simulink model "power_aircraft_distribution"  (R2014b)
settings: Solver=ode4  StartTime=0.0  StopTime=4.5  FixedStep=Ts  RelTol=5e-3
PreLoadFcn:
  | warning off
  | Ts=10e-6;
InitFcn:
  | warning off
  | Ts=10e-6;
StopFcn:
  | warning on
undefined symbols (not defined in the file or in its folder): D1, Delta, driveGuiManager, gcbh, sigbuilder_block
libraries: powerlib x51, simulink x4, simulink_extras x4, AC6DriveInternalModels x3, powerlib_meascontrol x2, DriveInternalModels x1, sps_avr x1
(part 1 of 2)
Description:
  | Copyright 2008-2014 The MathWorks, Inc.
settings Model: FPTRunName=Active  Creator=MathWorks  LastModifiedBy=JPSOLIV
settings SolverCC: MaxOrder=2  InsertRTBMode=Auto
settings DataIOCC: LimitDataPoints=off  SignalLoggingSaveFormat=ModelDataLogs  SaveOutput=off  SaveTime=off
settings OptimizationCC: ExpressionDepthLimit=2147483647  RollThreshold=1  InitFltsAndDblsToZero=on
settings DebuggingCC: SaveWithParameterizedLinksMsg=none  UnderspecifiedInitializationDetection=Classic  MergeDetectMultiDrivingBlocksExec=none  SignalResolutionControl=TryResolveAllWithWarning  MultiTaskDSMMsg=warning  MultiTaskCondExecSysMsg=none  MultiTaskRateTransMsg=warning  FcnCallInpInsideContextMsg=UseLocalSettings  StateNameClashWarn=warning
settings HardwareCC: TargetLongLongMode=on  TargetEndianess=LittleEndian  TargetHWDeviceType=MATLAB Host  ProdEqTarget=off
settings RTWCC: IncludeERTFirstTime=on
settings GRTTargetCC: TargetFcnLib=ansi_tfl_tmw.mat  CombineOutputUpdateFcns=off  GRTInterface=on

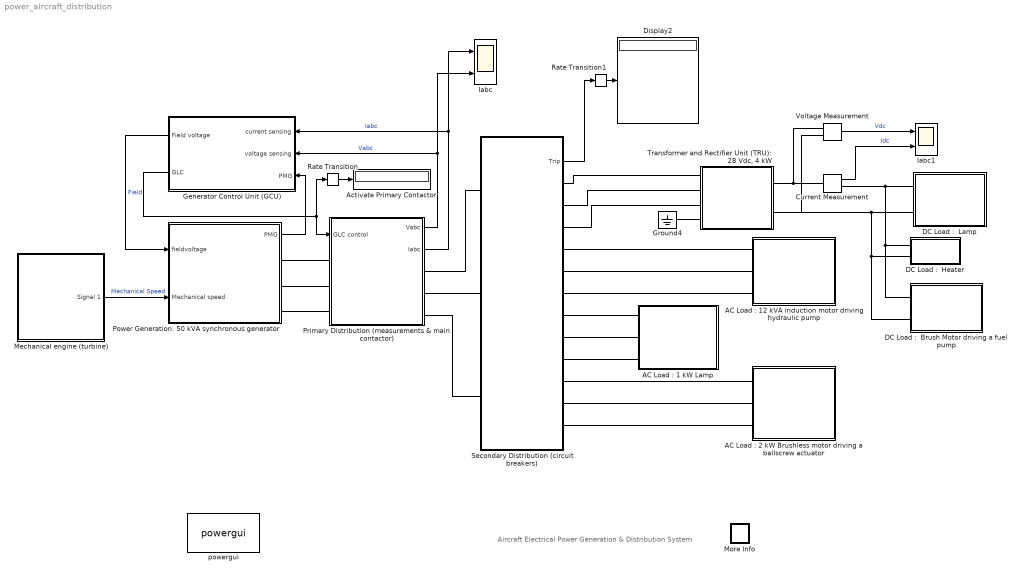
== system power_aircraft_distribution ==
  note: Aircraft Electrical Power Generation & Distribution System
  "AC Load : 1 kW Lamp" : Subsystem
      mask Display: image(imread('power_aircraft_distribution_ACLamp.jpg','jpg'))
  "AC Load : 12 kVA induction motor driving hydraulic pump" : Subsystem
      mask Display: image(imread('power_aircraft_distribution_EnginePump.jpg','jpg'))
  "AC Load : 2 kW Brushless motor driving a ballscrew actuator" : Subsystem
      mask Display: image(imread('power_aircraft_distribution_ballscrew.jpg','jpg'))
  Activate Primary Contactor : Display
      settings: SampleTime=1e-2
  Current Measurement : powerlib/Measurements/Current Measurement  PhasorSimulation=off  OutputType=Complex  PSBequivalent=0
  "DC Load :  Brush Motor driving a fuel pump" : Subsystem
      mask Display: image(imread('power_aircraft_distribution_FuelPump.jpg','jpg'))
  "DC Load :  Heater" : Subsystem
      mask Display: image(imread('power_aircraft_distribution_heater.jpg','jpg'))
  "DC Load :  Lamp" : Subsystem
      mask Display: image(imread('power_aircraft_distribution_DCLamp.jpg','jpg'))
  Display2 : Display
      settings: SampleTime=1e-2
  Generator Control Unit (GCU) : Subsystem
      mask Display: image(imread('power_aircraft_distribution_GCU.jpg','jpg'))
  Ground4 : powerlib/Elements/Ground  LConnTagsString=a
  Iabc : Scope  NumInputPorts=2
      settings: YMin=-5~-5  YMax=5~5
  Iabc1 : Scope  NumInputPorts=2
      settings: YMin=-5~-5  YMax=5~5
  Mechanical engine (turbine) : Subsystem  Tag=STV Subsys  LoadFcn=sigbuilder_block('load');  StartFcn=sigbuilder_block('start');  StopFcn=sigbuilder_block('stop');  ClipboardFcn=sigbuilder_block('clipboard');  mask(Sigbuilder block){}
      mask help: Sigbuilder GUI
      mask init:
      | if ~strcmp(get_param(bdroot(gcbh),'SimulationStatus'),'stopped') tuvar = sigbuilder_block('maskInit'); end
      settings: CopyFcn=sigbuilder_block('copy');  DeleteFcn=sigbuilder_block('delete');  ModelCloseFcn=sigbuilder_block('modelClose');  PreSaveFcn=sigbuilder_block('preSave');  PauseFcn=sigbuilder_block('pause')  ContinueFcn=sigbuilder_block('continue')  NameChangeFcn=sigbuilder_block('namechange');  OpenFcn=sigbuilder_block('open',[3 22.5 1194 819 ]);  CloseFcn=sigbuilder_block('close');
      mask Display: image(imread('power_aircraft_distribution_turbine.jpg','jpg'))
  More Info : Subsystem
      settings: OpenFcn=showdemo(bdroot(gcb))
      mask Display: disp('?')
  Power Generation: 50 kVA synchronous generator : Subsystem
      mask Display: image(imread('power_aircraft_distribution_APU_Generator.jpg','jpg'))
  Primary Distribution (measurements & main contactor) : Subsystem
  Rate Transition : RateTransition  OutPortSampleTimeOpt=Inherit  OutPortSampleTime=Ts
  Rate Transition1 : RateTransition  OutPortSampleTimeOpt=Inherit  OutPortSampleTime=Ts
  Secondary Distribution (circuit breakers) : Subsystem  mask{FuseA=25, FuseB=200, FuseC=5, FuseD=30}
      mask prompts: FuseA "Breaker  TRU (Amps RMS)"; FuseB "Breaker AC motor (Amps RMS)"; FuseC "Breaker Lamp (Amps RMS)"; FuseD "Breaker Brushless (Amps RMS)"
  "Transformer and Rectifier Unit (TRU): 28 Vdc, 4 kW" : Subsystem
      mask Display: image(imread('power_aircraft_distribution_TRU.jpg','jpg'))
  Voltage Measurement : powerlib/Measurements/Voltage Measurement  PhasorSimulation=off  OutputType=Complex  PSBequivalent=0
  powergui : powerlib/powergui  SimulationMode=Discrete  SolverType=Tustin/Backward Euler (TBE)  SampleTime=Ts  frequency=60  SPID=off  DisableSnubberDevices=off  DisableRonSwitches=off  DisableVfSwitches=off  SwTol=0  DisplayEquations=off  Interpol=off  methode=off  Ts=0  frequencyindice=0  Pbase=100e6  ErrMax=1e-4  Iterations=50  UnitsV=kV  UnitsW=MW  FunctionMessages=off  echomessages=off  HookPort=off  EnableUseOfTLC=off  x0status=blocks  RestoreLinks=no  ResistiveCurrentMeasurement=off  Frange=[0:2:500]  Ylog=off  Xlog=on  ShowGrid=off  save=off  variable=ZData  structure=0  ZoomFFT=on  StartTime=0.0  cycles=1  DisplayStyle=1  fundamental=60  FreqAxis=off  MaxFrequency=1000  frequencyindicesteady=1  RmsSteady=1  display=off
  wires:
  Power Generation: 50 kVA synchronous generator/1(PMG) -> Generator Control Unit (GCU)/3(PMG)
  Generator Control Unit (GCU)/1(Field voltage) -> Power Generation: 50 kVA synchronous generator/1(fieldvoltage)  "Field"
  Primary Distribution (measurements & main contactor)/1(Vabc) -> Generator Control Unit (GCU)/2(voltage sensing), Iabc/2  "Vabc"
  Primary Distribution (measurements & main contactor)/2(Iabc) -> Iabc/1, Generator Control Unit (GCU)/1(current sensing)  "Iabc"
  Generator Control Unit (GCU)/2(GLC) -> Primary Distribution (measurements & main contactor)/1(GLC control), Rate Transition/1
  Secondary Distribution (circuit breakers)/1(Trip) -> Rate Transition1/1
  Mechanical engine (turbine)/1(Signal 1) -> Power Generation: 50 kVA synchronous generator/2(Mechanical speed)  "Mechanical Speed"
  Current Measurement/1 -> Iabc1/2  "Idc"
  Voltage Measurement/1 -> Iabc1/1  "Vdc"
  Rate Transition/1 -> Activate Primary Contactor/1
  Rate Transition1/1 -> Display2/1
  connections:
  Power Generation: 50 kVA synchronous generator/RConn1 -- Primary Distribution (measurements & main contactor)/LConn1
  Power Generation: 50 kVA synchronous generator/RConn2 -- Primary Distribution (measurements & main contactor)/LConn2
  Power Generation: 50 kVA synchronous generator/RConn3 -- Primary Distribution (measurements & main contactor)/LConn3
  Primary Distribution (measurements & main contactor)/RConn1 -- Secondary Distribution (circuit breakers)/LConn1
  Secondary Distribution (circuit breakers)/LConn2 -- Primary Distribution (measurements & main contactor)/RConn2
  Secondary Distribution (circuit breakers)/LConn3 -- Primary Distribution (measurements & main contactor)/RConn3
  Secondary Distribution (circuit breakers)/RConn5 -- "AC Load : 12 kVA induction motor driving hydraulic pump"/LConn2
  Secondary Distribution (circuit breakers)/RConn6 -- "AC Load : 12 kVA induction motor driving hydraulic pump"/LConn3
  Secondary Distribution (circuit breakers)/RConn12 -- "AC Load : 2 kW Brushless motor driving a ballscrew actuator"/LConn3
  Secondary Distribution (circuit breakers)/RConn10 -- "AC Load : 2 kW Brushless motor driving a ballscrew actuator"/LConn1
  Secondary Distribution (circuit breakers)/RConn4 -- "AC Load : 12 kVA induction motor driving hydraulic pump"/LConn1
  Ground4/LConn1 -- "Transformer and Rectifier Unit (TRU): 28 Vdc, 4 kW"/LConn4
  Secondary Distribution (circuit breakers)/RConn11 -- "AC Load : 2 kW Brushless motor driving a ballscrew actuator"/LConn2
  "DC Load :  Lamp"/LConn1 -- "DC Load :  Heater"/LConn1 -- "DC Load :  Brush Motor driving a fuel pump"/LConn1 -- Current Measurement/RConn1
  "Transformer and Rectifier Unit (TRU): 28 Vdc, 4 kW"/RConn1 -- Current Measurement/LConn1 -- Voltage Measurement/LConn1
  "DC Load :  Heater"/LConn2 -- "DC Load :  Brush Motor driving a fuel pump"/LConn2 -- Voltage Measurement/LConn2 -- "Transformer and Rectifier Unit (TRU): 28 Vdc, 4 kW"/RConn2 -- "DC Load :  Lamp"/LConn2
  Secondary Distribution (circuit breakers)/RConn1 -- "Transformer and Rectifier Unit (TRU): 28 Vdc, 4 kW"/LConn1
  Secondary Distribution (circuit breakers)/RConn2 -- "Transformer and Rectifier Unit (TRU): 28 Vdc, 4 kW"/LConn2
  Secondary Distribution (circuit breakers)/RConn3 -- "Transformer and Rectifier Unit (TRU): 28 Vdc, 4 kW"/LConn3
  Secondary Distribution (circuit breakers)/RConn7 -- "AC Load : 1 kW Lamp"/LConn1
  Secondary Distribution (circuit breakers)/RConn8 -- "AC Load : 1 kW Lamp"/LConn2
  Secondary Distribution (circuit breakers)/RConn9 -- "AC Load : 1 kW Lamp"/LConn3

== system power_aircraft_distribution/AC Load : 1 kW Lamp ==
  note: AC Load
  Lamp 1000 Watts : powerlib/Elements/Three-Phase Series RLC Load  LConnTagsString=A|B|C  Configuration=Y (grounded)  NominalVoltage=200  NominalFrequency=400  ActivePower=1000  InductivePower=0  CapacitivePower=0  Measurements=None  LoadType=constant Z
  A : PMIOPort  Port=1  Side=Left
  B : PMIOPort  Port=2  Side=Left
  C : PMIOPort  Port=3  Side=Left
  connections:
  A/RConn1 -- Lamp 1000 Watts/LConn1
  B/RConn1 -- Lamp 1000 Watts/LConn2
  C/RConn1 -- Lamp 1000 Watts/LConn3

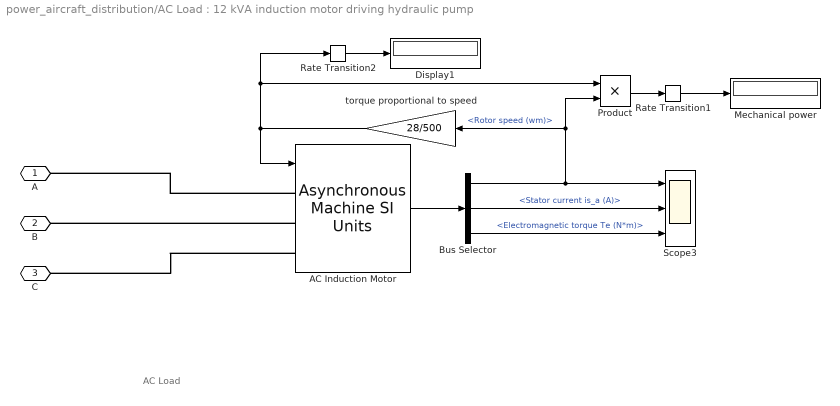
== system power_aircraft_distribution/AC Load : 12 kVA induction motor driving hydraulic pump ==
  note: AC Load
  AC Induction Motor : powerlib/Machines/Asynchronous Machine SI Units  PresetModel=No  MechanicalLoad=Torque Tm  ShowDetailedParameters=on  RotorType=Squirrel-cage  ReferenceFrame=Rotor  Units=SI  MeasurementBus=off  NominalParameters=[12e3 200 400]  Stator=[0.2761 0.002191/10]  Rotor=[0.16 0.002191/10]  Cage1=[ 0.022 0.226/377]  Cage2=[ 0.022 0.226/377]  Lm=0.07614  Mechanical=[0.01 0 8]  PolePairs=8  InitialConditions=[1,0 0,0,0 0,0,0]  SimulateSaturation=off  Saturation=[14.03593122, 27.81365428, 53.79336849, 72.68890987, 97.98006896, 148.6815601, 215.7428561, 302.9841135, 428.7778367 ; 230, 322, 414, 460, 506, 552, 598, 644, 690]  LoadFlowParameters=0  TsPowergui=0  TsBlock=-1  IterativeModel=Trapezoidal non iterative  Pmec=0
  Bus Selector : BusSelector  OutputSignals=Mechanical.Rotor speed (wm),Stator measurements.Stator current is_a (A),Mechanical.Electromagnetic torque Te (N*m)
  Display1 : Display
      settings: SampleTime=1e-2
  Mechanical power : Display
      settings: SampleTime=1e-2
  Product : Product  RndMeth=Zero
  Rate Transition1 : RateTransition  OutPortSampleTimeOpt=Inherit  OutPortSampleTime=Ts
  Rate Transition2 : RateTransition  OutPortSampleTimeOpt=Inherit  OutPortSampleTime=Ts
  Scope3 : Scope  NumInputPorts=3
  torque proportional to speed : Gain  Gain=28/500
  A : PMIOPort  Port=1  Side=Left
  B : PMIOPort  Port=2  Side=Left
  C : PMIOPort  Port=3  Side=Left
  wires:
  AC Induction Motor/1 -> Bus Selector/1
  Bus Selector/1 -> Scope3/1, torque proportional to speed/1, Product/2  "<Rotor speed (wm)>"
  torque proportional to speed/1 -> AC Induction Motor/1, Product/1, Rate Transition2/1
  Product/1 -> Rate Transition1/1
  Bus Selector/2 -> Scope3/2  "<Stator current is_a (A)>"
  Bus Selector/3 -> Scope3/3  "<Electromagnetic torque Te (N*m)>"
  Rate Transition1/1 -> Mechanical power/1
  Rate Transition2/1 -> Display1/1
  connections:
  AC Induction Motor/LConn2 -- B/RConn1
  AC Induction Motor/LConn1 -- A/RConn1
  AC Induction Motor/LConn3 -- C/RConn1

== system power_aircraft_distribution/AC Load : 2 kW Brushless motor driving a ballscrew actuator ==
  note: AC Load
  Gain : Gain  Gain=0.2
  Line inductor : powerlib/Elements/Three-Phase Series RLC Branch  LConnTagsString=A|B|C  RConnTagsString=A|B|C  BranchType=L  Resistance=[]  Inductance=1e-3  Capacitance=[]  Measurements=None
  PM Synchronous Motor Drive1 : Subsystem  LoadFcn=driveGuiManager('Load',get_param(gcb,'driveType'), gcbh);  mask(PM Synchronous Motor Drive){AverageValue=on, MechanicalLoad=Torque Tm, driveType=AC6}
      mask prompts: AverageValue "Average value model"; MechanicalLoad "Mechanical input:"; driveType "Drive type:"
      mask init:
      | block = gcbh;
      | [X1,X1m,X2,X2m,X3,X4,Y1,Y1m,Y2,Y2m,Y3,Y4,color1,color2]=spsdrivelogo;
      | Ts = drivelibInitSampleTime(block);    
      | driveGuiManager('Siminit',driveType,block);
      | SetInternalDriveModel(driveType,AverageValue,block);
      | setInternalDriveMechInput(driveType,getfullname(block));
      | power_initmask();
      settings: DeleteFcn="driveGuiManager('Delete',get_param(gcb,'driveType')  ,gcbh)"  CloseFcn="driveGuiManager('Delete',get_param(gcb,'driveType')  ,gcbh)"  ParentCloseFcn="driveGuiManager('Hide',get_param(gcb,'driveType')  ,gcbh)"
      settings: OpenFcn=|
      | if (power_openblockproxy ('secondary'))
      | driveGuiManager('Create',get_param(gcb,'driveType')  ,gcbh)
      | end;
      mask Help: helpview(psbhelp)
      mask TypeOptions MechanicalLoad: Torque Tm | Speed w
      mask TypeOptions driveType: AC6
      mask Display:
      | patch([X1 X1m],[Y1 Y1m],color1);
      | patch(X3,Y3,color2);
      | plot([X1 X1m X2 X2m X3 X4],[Y1 Y1m Y2 Y2m Y3 Y4]);
      | text(0.5,0.3,'AC6','HorizontalAlignment','center')
  Scope : Scope  NumInputPorts=4
  Speed : powerlib_meascontrol/Pulse & Signal Generators/Stair Generator  t=[0 1.4 1.9 2.4 3]  e=[0 500 0 -500 0]  Ts=Ts
  demux : Subsystem
  A : PMIOPort  Port=1  Side=Left
  B : PMIOPort  Port=2  Side=Left
  C : PMIOPort  Port=3  Side=Left
  wires:
  Speed/1 -> PM Synchronous Motor Drive1/1(SP)
  Gain/1 -> PM Synchronous Motor Drive1/2(Tm)
  demux/1(i_a) -> Scope/1  "Stator current"
  demux/2(speed) -> Scope/2  "Rotor speed"
  demux/3(Tem) -> Scope/3  "Electromagnetic Torque"
  demux/4(v_dc) -> Scope/4  "DC bus voltage"
  PM Synchronous Motor Drive1/4(Wm) -> Gain/1
  PM Synchronous Motor Drive1/1(Motor) -> demux/1(motor)
  PM Synchronous Motor Drive1/2(Conv.) -> demux/2(Conv.)
  PM Synchronous Motor Drive1/3(Ctrl) -> demux/3(Ctrl)
  connections:
  Line inductor/RConn3 -- PM Synchronous Motor Drive1/LConn3
  Line inductor/RConn2 -- PM Synchronous Motor Drive1/LConn2
  Line inductor/RConn1 -- PM Synchronous Motor Drive1/LConn1
  Line inductor/LConn3 -- C/RConn1
  Line inductor/LConn2 -- B/RConn1
  Line inductor/LConn1 -- A/RConn1

== system power_aircraft_distribution/DC Load :  Brush Motor driving a fuel pump ==
  note: DC Load
  Bus Selector : BusSelector  OutputSignals=Speed wm (rad/s),Armature current ia (A),Electrical torque Te (n m)
  DC Machine : powerlib/Machines/DC Machine  PresetModel=No  MechanicalLoad=Torque TL  FieldType=Wound  ShowDetailedParameters=on  MeasurementBus=off  RLa=[ .35 0.0001]  RLf="[ 240  12]"  Laf=1  MachineConstant=Torque constant (N.m/A)  Ke=1.8  Kt=1.8  J=0.0005  Bm=0  Tf=0  w0=0  Ifinit=0  TsPowergui=0  TsBlock=-1
  Gain : Gain  Gain=1.5/200
  Scope3 : Scope  NumInputPorts=3
  + : PMIOPort  Port=1  Side=Left
  - : PMIOPort  Port=2  Side=Left
  wires:
  Gain/1 -> DC Machine/1
  DC Machine/1 -> Bus Selector/1
  Bus Selector/1 -> Scope3/1, Gain/1  "<Speed wm (rad/s)>"
  Bus Selector/2 -> Scope3/2  "<Armature current ia (A)>"
  Bus Selector/3 -> Scope3/3  "<Electrical torque Te (n m)>"
  connections:
  -/RConn1 -- DC Machine/RConn1 -- DC Machine/RConn2
  +/RConn1 -- DC Machine/LConn1 -- DC Machine/LConn2

== system power_aircraft_distribution/DC Load :  Heater ==
  note: DC Load
  Series RLC Branch3 : powerlib/Elements/Series RLC Branch  LConnTagsString=__new0  RConnTagsString=__new0  BranchType=R  Resistance=1  Inductance=[]  SetiL0=off  InitialCurrent=0  Capacitance=[]  Setx0=off  InitialVoltage=0  Measurements=Branch voltage and current
  + : PMIOPort  Port=1  Side=Left
  - : PMIOPort  Port=2  Side=Left
  connections:
  -/RConn1 -- Series RLC Branch3/RConn1
  +/RConn1 -- Series RLC Branch3/LConn1

== system power_aircraft_distribution/DC Load :  Lamp ==
  note: DC Load
  Series RLC Branch3 : powerlib/Elements/Series RLC Branch  LConnTagsString=__new0  RConnTagsString=__new0  BranchType=R  Resistance=1  Inductance=[]  SetiL0=off  InitialCurrent=0  Capacitance=[]  Setx0=off  InitialVoltage=0  Measurements=Branch voltage and current
  + : PMIOPort  Port=1  Side=Left
  - : PMIOPort  Port=2  Side=Left
  connections:
  +/RConn1 -- Series RLC Branch3/LConn1
  -/RConn1 -- Series RLC Branch3/RConn1

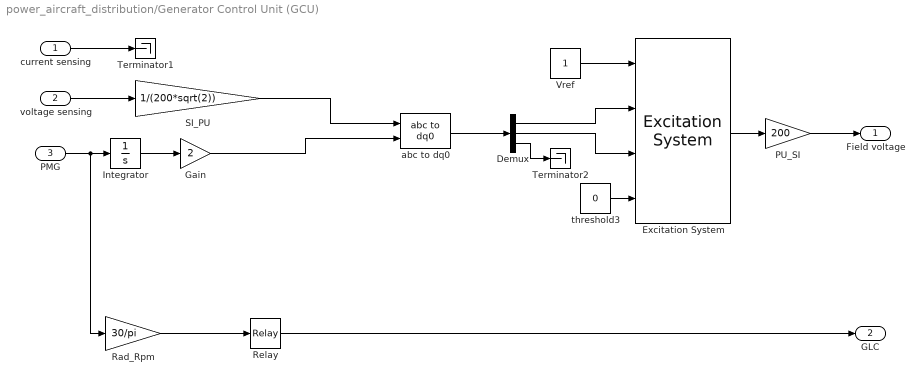
== system power_aircraft_distribution/Generator Control Unit (GCU) ==
  current sensing : Inport
  voltage sensing : Inport  Port=2
  PMG : Inport  Port=3
  Demux : Demux  Outputs=3
  Excitation System : sps_avr/Excitation System  tr=20e-3  reg=[ 300, 0.001 ]  exc=[ 1, 0 ]  tgr=[ 0, 0 ]  damp=[ 0.001, 0.1 ]  sat=[ 0, 0 ]  lim=[ -2, 2, 0 ]  v0=[1 0]
  Gain : Gain  Gain=2
  Integrator : Integrator
  PU_SI : Gain  Gain=200
  Rad_Rpm : Gain  Gain=30/pi
  Relay : Relay  OnSwitchValue=9000  OffSwitchValue=8900
  SI_PU : Gain  Gain=1/(200*sqrt(2))
  Terminator1 : Terminator
  Terminator2 : Terminator
  Vref : Constant
  abc to dq0 : powerlib_meascontrol/Transformations/abc to dq0  Alignment=90 degrees behind phase A axis
  threshold3 : Constant  Value=0
  Field voltage : Outport
  GLC : Outport  Port=2
  wires:
  Relay/1 -> GLC/1
  Demux/3 -> Terminator2/1
  current sensing/1 -> Terminator1/1
  threshold3/1 -> Excitation System/4
  Vref/1 -> Excitation System/1
  Rad_Rpm/1 -> Relay/1
  PU_SI/1 -> Field voltage/1
  Excitation System/1 -> PU_SI/1
  SI_PU/1 -> abc to dq0/1
  Demux/2 -> Excitation System/3
  Demux/1 -> Excitation System/2
  abc to dq0/1 -> Demux/1
  Integrator/1 -> Gain/1
  voltage sensing/1 -> SI_PU/1
  PMG/1 -> Rad_Rpm/1, Integrator/1
  Gain/1 -> abc to dq0/2

== system power_aircraft_distribution/Mechanical engine (turbine) ==
  Demux : Demux  Tag=STV Demux  Outputs=1
  FromWs : FromWorkspace  Tag=STV FromWs  VariableName=tuvar  SampleTime=0
      SigBuilderData=|
      | common.afterFinalStr = 'Extrapolate'
      | common.sampleTime = 0
      | dataSet.timeRange = [0 10]
      | dataSet.name = 'Group 1'
      | sbobj.Groups.Name = 'Group 1'
      | sbobj.Groups.Signals.Name = 'Signal 1'
      | sbobj.Groups.Signals.XData = [0 0.4 0.5 1 2 3 4.5 6 6 10]
      | sbobj.Groups.Signals.YData = [0 12000 12000 12000 12000 10000 18000 1 0 0]
  Signal 1 : Outport  Tag=STV Outport
  wires:
  FromWs/1 -> Demux/1
  Demux/1 -> Signal 1/1

== system power_aircraft_distribution/More Info ==

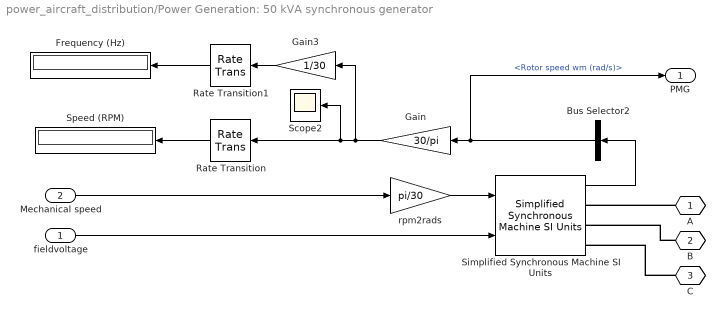
== system power_aircraft_distribution/Power Generation: 50 kVA synchronous generator ==
  fieldvoltage : Inport
  Mechanical speed : Inport  Port=2
  Bus Selector2 : BusSelector  OutputSignals=Rotor speed wm (rad/s)
  Frequency (Hz) : Display
      settings: SampleTime=1e-2
  Gain : Gain  Gain=30/pi
  Gain3 : Gain  Gain=1/30
  Rate Transition : RateTransition  OutPortSampleTimeOpt=Inherit  OutPortSampleTime=Ts
  Rate Transition1 : RateTransition  OutPortSampleTimeOpt=Inherit  OutPortSampleTime=Ts
  Scope2 : Scope
  Simplified Synchronous Machine SI Units : powerlib/Machines/Simplified Synchronous Machine SI Units  ConnectionType=3-wire Y  MechanicalLoad=Speed w  MeasurementBus=off  NominalParameters=[50e3 200 400]  Mechanical=[0.02 0 2]  InternalRL="[0.0204  0.08104e-3]"  InitialConditions=[-99,0 0,0,0 0,0,0]  Units=1  LoadFlowParameters=[1,0,0,0,0]  TsPowergui=0  TsBlock=Ts  BusType=PV  Pref=0  Qref=0  Qmin=-inf  Qmax=+inf  PLF=0  QLF=0
  Speed (RPM) : Display
      settings: SampleTime=1e-2
  rpm2rads : Gain  Gain=pi/30
  A : PMIOPort  Tag=PMCPort  Port=1  Side=Right
  B : PMIOPort  Tag=PMCPort  Port=2  Side=Right
  C : PMIOPort  Tag=PMCPort  Port=3  Side=Right
  PMG : Outport
  wires:
  Simplified Synchronous Machine SI Units/1 -> Bus Selector2/1
  fieldvoltage/1 -> Simplified Synchronous Machine SI Units/2
  Bus Selector2/1 -> Gain/1, PMG/1  "<Rotor speed wm (rad/s)>"
  Gain/1 -> Gain3/1, Scope2/1, Rate Transition/1
  Gain3/1 -> Rate Transition1/1
  Mechanical speed/1 -> rpm2rads/1
  rpm2rads/1 -> Simplified Synchronous Machine SI Units/1
  Rate Transition/1 -> Speed (RPM)/1
  Rate Transition1/1 -> Frequency (Hz)/1
  connections:
  A/RConn1 -- Simplified Synchronous Machine SI Units/RConn1
  B/RConn1 -- Simplified Synchronous Machine SI Units/RConn2
  C/RConn1 -- Simplified Synchronous Machine SI Units/RConn3

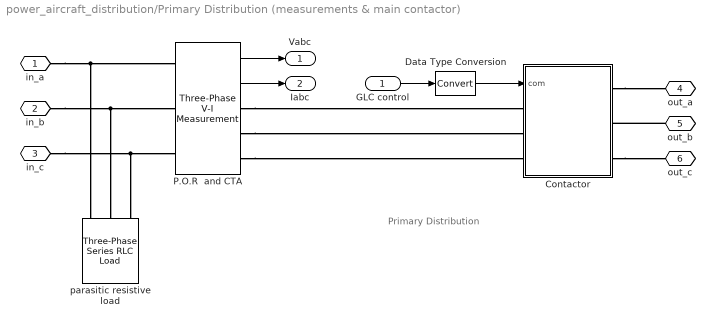
== system power_aircraft_distribution/Primary Distribution (measurements & main contactor) ==
  note: Primary Distribution
  GLC control : Inport
  Contactor : Subsystem
  Data Type Conversion : DataTypeConversion
  P.O.R  and CTA : powerlib/Measurements/Three-Phase V-I Measurement  VoltageMeasurement=phase-to-phase  SetLabelV=off  LabelV=Vabc  Vpu=off  VpuLL=off  CurrentMeasurement=yes  SetLabelI=off  LabelI=Iabc  Ipu=off  Pbase=100e6  Vbase=500e3  OutputType=Complex  PhasorSimulation=off  PSBequivalent=0
  parasitic resistive load : powerlib/Elements/Three-Phase Series RLC Load  LConnTagsString=A|B|C  Configuration=Y (grounded)  NominalVoltage=200  NominalFrequency=400  ActivePower=5000  InductivePower=0  CapacitivePower=0  Measurements=None  LoadType=constant Z
  in_a : PMIOPort  Port=1  Side=Left
  in_b : PMIOPort  Port=2  Side=Left
  in_c : PMIOPort  Port=3  Side=Left
  out_a : PMIOPort  Port=4  Side=Right
  out_b : PMIOPort  Port=5  Side=Right
  out_c : PMIOPort  Port=6  Side=Right
  Vabc : Outport
  Iabc : Outport  Port=2
  wires:
  GLC control/1 -> Data Type Conversion/1
  P.O.R  and CTA/1 -> Vabc/1
  P.O.R  and CTA/2 -> Iabc/1
  Data Type Conversion/1 -> Contactor/1(com)
  connections:
  in_a/RConn1 -- P.O.R  and CTA/LConn1 -- parasitic resistive load/LConn1
  in_b/RConn1 -- P.O.R  and CTA/LConn2 -- parasitic resistive load/LConn2
  in_c/RConn1 -- P.O.R  and CTA/LConn3 -- parasitic resistive load/LConn3
  P.O.R  and CTA/RConn1 -- Contactor/LConn1
  P.O.R  and CTA/RConn2 -- Contactor/LConn2
  P.O.R  and CTA/RConn3 -- Contactor/LConn3
  Contactor/RConn1 -- out_a/RConn1
  out_b/RConn1 -- Contactor/RConn2
  Contactor/RConn3 -- out_c/RConn1

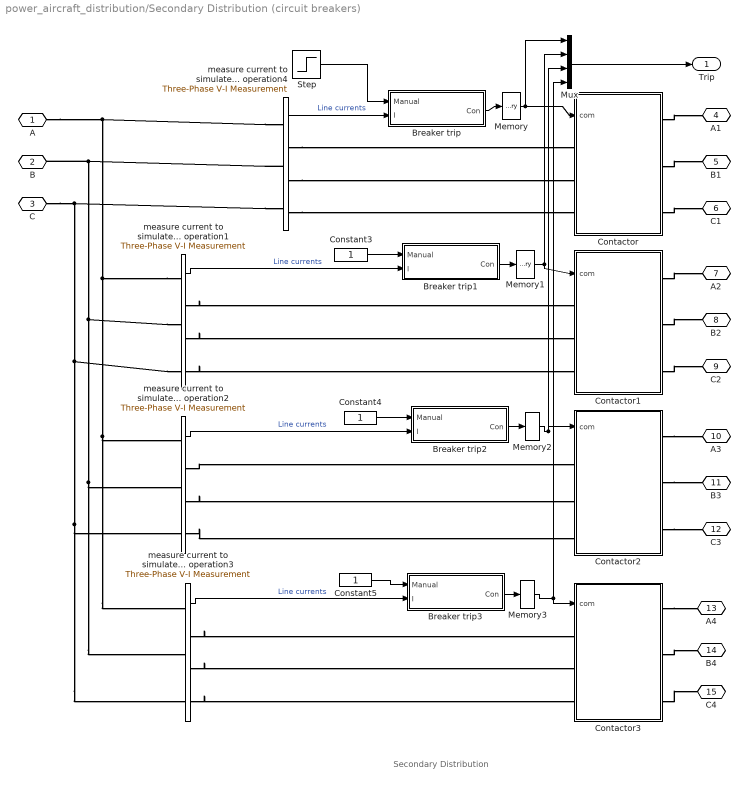
== system power_aircraft_distribution/Secondary Distribution (circuit breakers) ==
  note: Secondary Distribution
  Breaker trip : Subsystem
  Breaker trip1 : Subsystem
  Breaker trip2 : Subsystem
  Breaker trip3 : Subsystem
  Constant3 : Constant  OutDataTypeStr=boolean
  Constant4 : Constant  OutDataTypeStr=boolean
  Constant5 : Constant  OutDataTypeStr=boolean
  Contactor : Subsystem
  Contactor1 : Subsystem
  Contactor2 : Subsystem
  Contactor3 : Subsystem
  Memory{,1..3} (4 alike) : Memory
  Mux : Mux
  Step : Step  Time=3.5  Before=1  After=0  SampleTime=0
  measure current to simulate fuse operation{1..4} (4 alike) : powerlib/Measurements/Three-Phase V-I Measurement  VoltageMeasurement=no  SetLabelV=off  LabelV=Vabc  Vpu=off  VpuLL=off  CurrentMeasurement=yes  SetLabelI=off  LabelI=Iabc  Ipu=off  Pbase=100e6  Vbase=500e3  OutputType=Complex  PhasorSimulation=off  PSBequivalent=0
  A : PMIOPort  Port=1  Side=Left
  B : PMIOPort  Port=2  Side=Left
  C : PMIOPort  Port=3  Side=Left
  A1 : PMIOPort  Port=4  Side=Right
  B1 : PMIOPort  Port=5  Side=Right
  C1 : PMIOPort  Port=6  Side=Right
  A2 : PMIOPort  Port=7  Side=Right
  B2 : PMIOPort  Port=8  Side=Right
  C2 : PMIOPort  Port=9  Side=Right
  A3 : PMIOPort  Port=10  Side=Right
  B3 : PMIOPort  Port=11  Side=Right
  C3 : PMIOPort  Port=12  Side=Right
  A4 : PMIOPort  Port=13  Side=Right
  B4 : PMIOPort  Port=14  Side=Right
  C4 : PMIOPort  Port=15  Side=Right
  Trip : Outport
  wires:
  Constant3/1 -> Breaker trip1/1(Manual)
  Step/1 -> Breaker trip/1(Manual)
  Memory3/1 -> Contactor3/1(com), Mux/4
  Memory2/1 -> Contactor2/1(com), Mux/3
  Breaker trip1/1(Con) -> Memory1/1
  Memory/1 -> Contactor/1(com), Mux/1
  Memory1/1 -> Contactor1/1(com), Mux/2
  Mux/1 -> Trip/1
  Breaker trip2/1(Con) -> Memory2/1
  Breaker trip3/1(Con) -> Memory3/1
  Constant4/1 -> Breaker trip2/1(Manual)
  Constant5/1 -> Breaker trip3/1(Manual)
  measure current to simulate fuse operation3/1 -> Breaker trip3/2(I)  "Line currents"
  measure current to simulate fuse operation2/1 -> Breaker trip2/2(I)  "Line currents"
  measure current to simulate fuse operation1/1 -> Breaker trip1/2(I)  "Line currents"
  Breaker trip/1(Con) -> Memory/1
  measure current to simulate fuse operation4/1 -> Breaker trip/2(I)  "Line currents"
  connections:
  measure current to simulate fuse operation3/RConn3 -- Contactor3/LConn3
  measure current to simulate fuse operation3/RConn2 -- Contactor3/LConn2
  measure current to simulate fuse operation3/RConn1 -- Contactor3/LConn1
  Contactor3/RConn3 -- C4/RConn1
  Contactor3/RConn2 -- B4/RConn1
  Contactor3/RConn1 -- A4/RConn1
  measure current to simulate fuse operation2/RConn3 -- Contactor2/LConn3
  measure current to simulate fuse operation2/RConn2 -- Contactor2/LConn2
  measure current to simulate fuse operation2/RConn1 -- Contactor2/LConn1
  Contactor2/RConn3 -- C3/RConn1
  Contactor2/RConn2 -- B3/RConn1
  Contactor2/RConn1 -- A3/RConn1
  measure current to simulate fuse operation1/RConn3 -- Contactor1/LConn3
  measure current to simulate fuse operation1/RConn2 -- Contactor1/LConn2
  measure current to simulate fuse operation1/RConn1 -- Contactor1/LConn1
  Contactor1/RConn3 -- C2/RConn1
  Contactor1/RConn2 -- B2/RConn1
  Contactor1/RConn1 -- A2/RConn1
  measure current to simulate fuse operation4/RConn3 -- Contactor/LConn3
  measure current to simulate fuse operation4/RConn2 -- Contactor/LConn2
  measure current to simulate fuse operation4/RConn1 -- Contactor/LConn1
  Contactor/RConn3 -- C1/RConn1
  Contactor/RConn2 -- B1/RConn1
  Contactor/RConn1 -- A1/RConn1
  measure current to simulate fuse operation1/LConn3 -- measure current to simulate fuse operation4/LConn3 -- C/RConn1 -- measure current to simulate fuse operation2/LConn3 -- measure current to simulate fuse operation3/LConn3
  measure current to simulate fuse operation1/LConn2 -- measure current to simulate fuse operation2/LConn2 -- measure current to simulate fuse operation3/LConn2 -- B/RConn1 -- measure current to simulate fuse operation4/LConn2
  measure current to simulate fuse operation1/LConn1 -- measure current to simulate fuse operation2/LConn1 -- measure current to simulate fuse operation3/LConn1 -- measure current to simulate fuse operation4/LConn1 -- A/RConn1

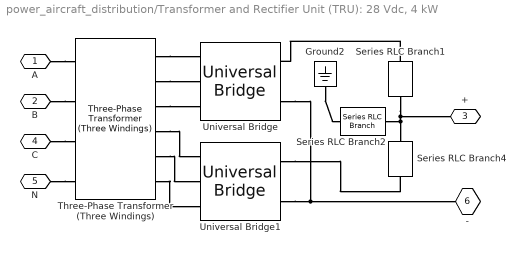
== system power_aircraft_distribution/Transformer and Rectifier Unit (TRU): 28 Vdc, 4 kW ==
  Ground2 : powerlib/Elements/Ground  LConnTagsString=a
  Series RLC Branch1 : powerlib/Elements/Series RLC Branch  LConnTagsString=__new0  RConnTagsString=__new0  BranchType=L  Resistance=[]  Inductance=2e-3  SetiL0=on  InitialCurrent=0  Capacitance=[]  Setx0=off  InitialVoltage=0  Measurements=Branch voltage and current
  Series RLC Branch2 : powerlib/Elements/Series RLC Branch  LConnTagsString=__new0  RConnTagsString=__new0  BranchType=C  Resistance=[]  Inductance=[]  SetiL0=off  InitialCurrent=0  Capacitance=1e-6  Setx0=off  InitialVoltage=0  Measurements=None
  Series RLC Branch4 : powerlib/Elements/Series RLC Branch  LConnTagsString=__new0  RConnTagsString=__new0  BranchType=L  Resistance=[]  Inductance=2e-3  SetiL0=off  InitialCurrent=0  Capacitance=[]  Setx0=off  InitialVoltage=0  Measurements=Branch voltage and current
  Three-Phase Transformer (Three Windings) : powerlib/Elements/Three-Phase Transformer (Three Windings)  Winding1Connection=Yn  UNITS=pu  NominalPower=[ 4200 , 600 ]  Winding1=[ 200 , 0.0002 , 0 ]  Winding2Connection=Delta (D1)  Winding2=[ 22 , 0.0002 , 0 ]  Winding3Connection=Delta (D1)  Winding3=[ 22 , 0.0002 , 0]  SetSaturation=off  Rm=500  Lm=500*10  Saturation=[ 0,0 ; 0.0024,1.2 ; 1.0,1.52 ]  Hysteresis=off  DataFile='hysteresis'  SetInitialFlux=off  InitialFluxes=[0.8 -0.8 0.7]  Measurements=None  MoreParameters=off  BreakLoop=off  DataType=off  TransfoNumber=0
  Universal Bridge : powerlib/Power Electronics/Universal Bridge  Arms=3  SnubberResistance=1e3  SnubberCapacitance=1e-6  Device=Diodes  Ron=1e-3  Lon=0  ForwardVoltages="[  0  0  ]"  ForwardVoltage=0.8  GTOparameters=[ 10e-6 , 20e-6 ]  IGBTparameters=[ 1e-6 , 2e-6 ]  Measurements=None  Measurements_2=None  converterType=Rectifier
  Universal Bridge1 : powerlib/Power Electronics/Universal Bridge  Arms=3  SnubberResistance=1e3  SnubberCapacitance=1e-6  Device=Diodes  Ron=1e-3  Lon=0  ForwardVoltages="[  0  0  ]"  ForwardVoltage=0.8  GTOparameters=[ 10e-6 , 20e-6 ]  IGBTparameters=[ 1e-6 , 2e-6 ]  Measurements=None  Measurements_2=None  converterType=Rectifier
  A : PMIOPort  Port=1  Side=Left
  B : PMIOPort  Port=2  Side=Left
  + : PMIOPort  Port=3  Side=Right
  C : PMIOPort  Port=4  Side=Left
  N : PMIOPort  Port=5  Side=Left
  - : PMIOPort  Port=6  Side=Right
  connections:
  Ground2/LConn1 -- Series RLC Branch2/RConn1
  Universal Bridge/RConn2 -- Universal Bridge1/RConn2 -- -/RConn1
  Three-Phase Transformer (Three Windings)/RConn1 -- Universal Bridge/LConn1
  Three-Phase Transformer (Three Windings)/RConn2 -- Universal Bridge/LConn2
  Three-Phase Transformer (Three Windings)/RConn3 -- Universal Bridge/LConn3
  A/RConn1 -- Three-Phase Transformer (Three Windings)/LConn1
  B/RConn1 -- Three-Phase Transformer (Three Windings)/LConn2
  C/RConn1 -- Three-Phase Transformer (Three Windings)/LConn3
  N/RConn1 -- Three-Phase Transformer (Three Windings)/LConn4
  Series RLC Branch1/LConn1 -- Universal Bridge/RConn1
  Series RLC Branch2/LConn1 -- Series RLC Branch1/RConn1 -- +/RConn1 -- Series RLC Branch4/LConn1
  Three-Phase Transformer (Three Windings)/RConn4 -- Universal Bridge1/LConn1
  Three-Phase Transformer (Three Windings)/RConn5 -- Universal Bridge1/LConn2
  Three-Phase Transformer (Three Windings)/RConn6 -- Universal Bridge1/LConn3
  Universal Bridge1/RConn1 -- Series RLC Branch4/RConn1

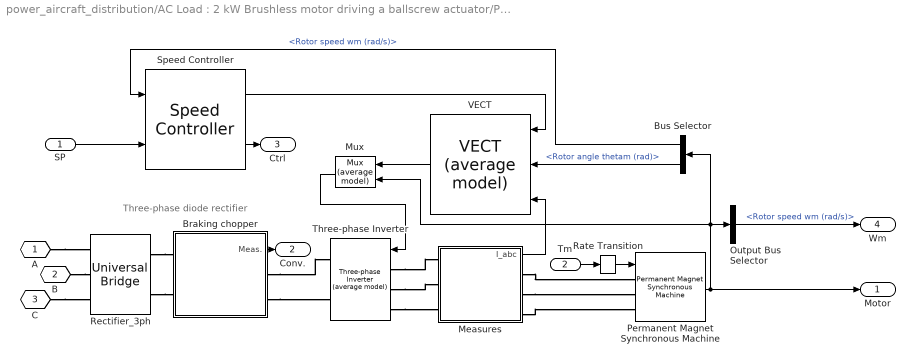
== system power_aircraft_distribution/AC Load : 2 kW Brushless motor driving a ballscrew actuator/PM Synchronous Motor Drive1 ==
  note: Three-phase
      | diode rectifier
  SP : Inport
  Tm : Inport  Port=2
  Braking chopper : Subsystem  StartFcn=|  mask(Braking chopper){chopa=290, chopd=280, freq_chop=4000, cap_bus=2000e-6, br=8}
      | chopa=str2num(get_param(gcb,'chopa'));                                                               
      | chopd=str2num(get_param(gcb,'chopd'));                                                               
      | if (chopa < chopd)                                                                                   
      |     error('Activation voltage must be greater than or equal to shutdown voltage in Braking chopper');
      | end
      mask prompts: chopa "Chopper activation voltage (V)"; chopd "Chopper shutdown voltage (V)"; freq_chop "Braking chopper frequency (Hz)"; cap_bus "DC bus capacitance (F)"; br "Braking resistance (ohms)"
      mask help: This block implement a DC link between the rectifier and the inverter. It also contains a DC bus integrated braking chopper. The braking resistor must be set properly to avoid oscillation.
      mask init:
      | if chopa < chopd;
      |     chopa = chopd;
      | end
      | [X1,X1m,X2,X2m,X3,X4,Y1,Y1m,Y2,Y2m,Y3,Y4,color1,color2]=spsdrivelogo;
      mask Display:
      | patch([X1 X1m],[Y1 Y1m],color1);
      | patch(X3,Y3,color2);
      | plot([X1 X1m X2 X2m X3 X4],[Y1 Y1m Y2 Y2m Y3 Y4]);
  Bus Selector : BusSelector  OutputSignals=Rotor speed wm (rad/s),Rotor angle thetam (rad)
  Measures : Subsystem
  Mux : AC6DriveInternalModels/Mux (average model)
  Output Bus Selector : BusSelector  OutputSignals=Rotor speed wm (rad/s)
  Permanent Magnet Synchronous Machine : powerlib/Machines/Permanent Magnet Synchronous Machine  NbPhases=3  FluxDistribution=Sinusoidal  RotorType=Round  MechanicalLoad=Torque Tm  PresetModel=No  ShowDetailedParameters=on  MeasurementBus=off  Resistance=0.2  Inductance=0  dqInductances=[8.5e-3,8.5e-3]  La=0.000835  MachineConstant=Flux linkage established by magnets (V.s)  Flux=0.175  VoltageCst=126.966  TorqueCst=1.05  Flat=0  Mechanical=[0.089,0.005,4]  PolePairs=4  InitialConditions=[0,0,0,0]  InitialConditions5ph=[0 0 0 0 0 0]  TsPowergui=0  TsBlock=-1  RefAngle=90 degrees behind phase A axis (modified Park)
      settings: AttributesFormatString=\n
  Rate Transition : RateTransition  OutPortSampleTime=Ts
  Rectifier_3ph : powerlib/Power Electronics/Universal Bridge  Arms=3  SnubberResistance=10e3  SnubberCapacitance=20e-9  Device=Diodes  Ron=1e-3  Lon=0  ForwardVoltages="[  0,  0  ]"  ForwardVoltage=1.3  GTOparameters=[ 10e-6, 20e-6 ]  IGBTparameters=[ 1e-6 , 2e-6 ]  Measurements=All voltages and currents  Measurements_2=None  converterType=Rectifier
  Speed Controller : DriveInternalModels/AC drives/Speed Controller AC67/Speed Controller  SwK=Speed regulation  ramp=[-1000,1000]  kp=5  ki=100  fc=100  ctrl_sat=[-50,50]  Tsc=150e-6
  Three-phase Inverter : AC6DriveInternalModels/Three-phase Inverter (average model)  Arms=3  SnubberResistance=5000  SnubberCapacitance=inf  Device=IGBT / Diodes  Ron=1e-3  Lon=0  ForwardVoltages=[0.8,0.8]  ForwardVoltage=0  GTOparameters=[0,0]  IGBTparameters=[1e-6,2e-6]  Measurements=All voltages and currents  converterType=Inverter  SourceFrequency=60  dqInductances=[8.5e-3,8.5e-3]  Flux=0.175  Resistance=0.2  p=4
  VECT : AC6DriveInternalModels/VECT (average model)  nb_p=4  lambda=0.175  freq_max=20e3  Ts_vect=50e-6  h=0.1
  A : PMIOPort  Port=1  Side=Left
  B : PMIOPort  Port=2  Side=Left
  C : PMIOPort  Tag=PMCPort  Port=3  Side=Left
  Motor : Outport
  Conv. : Outport  Port=2
  Ctrl : Outport  Port=3
  Wm : Outport  Port=4
  wires:
  Bus Selector/2 -> VECT/2  "<Rotor angle thetam (rad)>"
  Bus Selector/1 -> Speed Controller/1  "<Rotor speed wm (rad/s)>"
  Mux/1 -> Three-phase Inverter/1
  VECT/1 -> Mux/1
  Speed Controller/2 -> Ctrl/1
  Tm/1 -> Rate Transition/1
  Speed Controller/1 -> VECT/1
  Measures/1(I_abc) -> VECT/3
  Permanent Magnet Synchronous Machine/1 -> Output Bus Selector/1, Bus Selector/1, Mux/2, Motor/1
  SP/1 -> Speed Controller/2
  Braking chopper/1(Meas.) -> Conv./1
  Output Bus Selector/1 -> Wm/1  "<Rotor speed wm (rad/s)>"
  Rate Transition/1 -> Permanent Magnet Synchronous Machine/1
  connections:
  Three-phase Inverter/LConn3 -- Measures/LConn3
  Three-phase Inverter/LConn2 -- Measures/LConn2
  Three-phase Inverter/LConn1 -- Measures/LConn1
  C/RConn1 -- Rectifier_3ph/LConn3
  B/RConn1 -- Rectifier_3ph/LConn2
  Measures/RConn3 -- Permanent Magnet Synchronous Machine/LConn3
  Measures/RConn2 -- Permanent Magnet Synchronous Machine/LConn2
  Measures/RConn1 -- Permanent Magnet Synchronous Machine/LConn1
  Braking chopper/RConn2 -- Three-phase Inverter/RConn2
  A/RConn1 -- Rectifier_3ph/LConn1
  Rectifier_3ph/RConn1 -- Braking chopper/LConn1
  Rectifier_3ph/RConn2 -- Braking chopper/LConn2
  Braking chopper/RConn1 -- Three-phase Inverter/RConn1

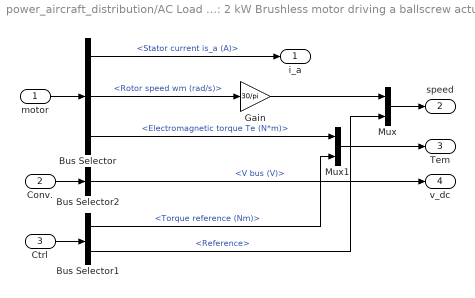
== system power_aircraft_distribution/AC Load : 2 kW Brushless motor driving a ballscrew actuator/demux ==
  motor : Inport
  Conv. : Inport  Port=2
  Ctrl : Inport  Port=3
  Bus Selector : BusSelector  OutputSignals=Stator current is_a (A),Rotor speed wm (rad/s),Electromagnetic torque Te (N*m)
  Bus Selector1 : BusSelector  OutputSignals=Torque reference (Nm),Reference
  Bus Selector2 : BusSelector  OutputSignals=V bus (V)
  Gain : Gain  Gain=30/pi  SaturateOnIntegerOverflow=on  OutDataTypeStr=Inherit: Same as input  ParamDataTypeStr=Inherit: Same as input
  Mux : Mux  Inputs=2
  Mux1 : Mux  Inputs=2
  i_a : Outport
  speed : Outport  Port=2
  Tem : Outport  Port=3
  v_dc : Outport  Port=4
  wires:
  Bus Selector/2 -> Gain/1  "<Rotor speed wm (rad/s)>"
  Bus Selector2/1 -> v_dc/1  "<V bus (V)>"
  Conv./1 -> Bus Selector2/1
  Ctrl/1 -> Bus Selector1/1
  Bus Selector1/1 -> Mux1/2  "<Torque reference (Nm)>"
  Bus Selector1/2 -> Mux/2  "<Reference>"
  Gain/1 -> Mux/1
  Bus Selector/1 -> i_a/1  "<Stator current is_a (A)>"
  Bus Selector/3 -> Mux1/1  "<Electromagnetic torque Te (N*m)>"
  Mux1/1 -> Tem/1
  Mux/1 -> speed/1
  motor/1 -> Bus Selector/1

== system power_aircraft_distribution/Primary Distribution (measurements & main contactor)/Contactor ==
  com : Inport
  Ideal Switch : powerlib/Power Electronics/Ideal Switch  Ron=0.001  Lon=0  IC=0  Rs=1e3  Cs=inf  Measurements=off
  Ideal Switch1 : powerlib/Power Electronics/Ideal Switch  Ron=0.001  Lon=0  IC=0  Rs=1e3  Cs=inf  Measurements=off
  Ideal Switch2 : powerlib/Power Electronics/Ideal Switch  Ron=0.001  Lon=0  IC=0  Rs=1e3  Cs=inf  Measurements=off
  A : PMIOPort  Port=1  Side=Left
  a : PMIOPort  Port=2  Side=Right
  B : PMIOPort  Port=3  Side=Left
  b : PMIOPort  Port=4  Side=Right
  C : PMIOPort  Port=5  Side=Left
  c : PMIOPort  Port=6  Side=Right
  wires:
  com/1 -> Ideal Switch1/1, Ideal Switch2/1, Ideal Switch/1
  connections:
  c/RConn1 -- Ideal Switch2/RConn1
  C/RConn1 -- Ideal Switch2/LConn1
  b/RConn1 -- Ideal Switch1/RConn1
  B/RConn1 -- Ideal Switch1/LConn1
  a/RConn1 -- Ideal Switch/RConn1
  A/RConn1 -- Ideal Switch/LConn1

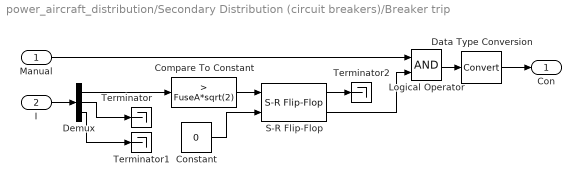
== system power_aircraft_distribution/Secondary Distribution (circuit breakers)/Breaker trip ==
  Manual : Inport
  I : Inport  Port=2
  Compare To Constant : simulink/Logic and Bit Operations/Compare To Constant  relop=>  const=FuseA*sqrt(2)  OutDataTypeStr=boolean  ZeroCross=off
  Constant : Constant  Value=0  OutDataTypeStr=boolean
  Data Type Conversion : DataTypeConversion
  Demux : Demux  Outputs=3
  Logical Operator : Logic  AllPortsSameDT=off  OutDataTypeStr=boolean
  S-R Flip-Flop : simulink_extras/Flip Flops/S-R Flip-Flop  initial_condition=0
  Terminator : Terminator
  Terminator1 : Terminator
  Terminator2 : Terminator
  Con : Outport
  wires:
  S-R Flip-Flop/2 -> Logical Operator/2
  S-R Flip-Flop/1 -> Terminator2/1
  Constant/1 -> S-R Flip-Flop/2
  Demux/3 -> Terminator1/1
  Demux/2 -> Terminator/1
  Compare To Constant/1 -> S-R Flip-Flop/1
  Data Type Conversion/1 -> Con/1
  Manual/1 -> Logical Operator/1
  Logical Operator/1 -> Data Type Conversion/1
  Demux/1 -> Compare To Constant/1
  I/1 -> Demux/1

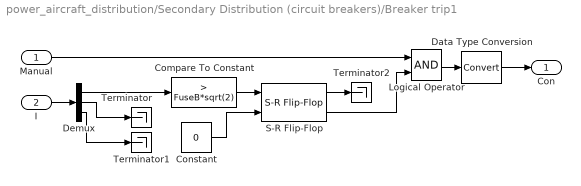
== system power_aircraft_distribution/Secondary Distribution (circuit breakers)/Breaker trip1 ==
  Manual : Inport
  I : Inport  Port=2
  Compare To Constant : simulink/Logic and Bit Operations/Compare To Constant  relop=>  const=FuseB*sqrt(2)  OutDataTypeStr=boolean  ZeroCross=off
  Constant : Constant  Value=0  OutDataTypeStr=boolean
  Data Type Conversion : DataTypeConversion
  Demux : Demux  Outputs=3
  Logical Operator : Logic  AllPortsSameDT=off  OutDataTypeStr=boolean
  S-R Flip-Flop : simulink_extras/Flip Flops/S-R Flip-Flop  initial_condition=0
  Terminator : Terminator
  Terminator1 : Terminator
  Terminator2 : Terminator
  Con : Outport
  wires:
  I/1 -> Demux/1
  Demux/1 -> Compare To Constant/1
  Logical Operator/1 -> Data Type Conversion/1
  Manual/1 -> Logical Operator/1
  Data Type Conversion/1 -> Con/1
  Compare To Constant/1 -> S-R Flip-Flop/1
  Demux/2 -> Terminator/1
  Demux/3 -> Terminator1/1
  Constant/1 -> S-R Flip-Flop/2
  S-R Flip-Flop/1 -> Terminator2/1
  S-R Flip-Flop/2 -> Logical Operator/2

== system power_aircraft_distribution/Secondary Distribution (circuit breakers)/Breaker trip2 ==
  Manual : Inport
  I : Inport  Port=2
  Compare To Constant : simulink/Logic and Bit Operations/Compare To Constant  relop=>  const=FuseC*sqrt(2)  OutDataTypeStr=boolean  ZeroCross=off
  Constant : Constant  Value=0  OutDataTypeStr=boolean
  Data Type Conversion : DataTypeConversion
  Demux : Demux  Outputs=3
  Logical Operator : Logic  AllPortsSameDT=off  OutDataTypeStr=boolean
  S-R Flip-Flop : simulink_extras/Flip Flops/S-R Flip-Flop  initial_condition=0
  Terminator : Terminator
  Terminator1 : Terminator
  Terminator2 : Terminator
  Con : Outport
  wires:
  S-R Flip-Flop/2 -> Logical Operator/2
  S-R Flip-Flop/1 -> Terminator2/1
  Constant/1 -> S-R Flip-Flop/2
  Demux/3 -> Terminator1/1
  Demux/2 -> Terminator/1
  Compare To Constant/1 -> S-R Flip-Flop/1
  Data Type Conversion/1 -> Con/1
  Manual/1 -> Logical Operator/1
  Logical Operator/1 -> Data Type Conversion/1
  Demux/1 -> Compare To Constant/1
  I/1 -> Demux/1

== system power_aircraft_distribution/Secondary Distribution (circuit breakers)/Breaker trip3 ==
  Manual : Inport
  I : Inport  Port=2
  Compare To Constant : simulink/Logic and Bit Operations/Compare To Constant  relop=>  const=FuseD*sqrt(2)  OutDataTypeStr=boolean  ZeroCross=off
  Constant : Constant  Value=0  OutDataTypeStr=boolean
  Data Type Conversion : DataTypeConversion
  Demux : Demux  Outputs=3
  Logical Operator : Logic  AllPortsSameDT=off  OutDataTypeStr=boolean
  S-R Flip-Flop : simulink_extras/Flip Flops/S-R Flip-Flop  initial_condition=0
  Terminator : Terminator
  Terminator1 : Terminator
  Terminator2 : Terminator
  Con : Outport
  wires:
  I/1 -> Demux/1
  Demux/1 -> Compare To Constant/1
  Logical Operator/1 -> Data Type Conversion/1
  Manual/1 -> Logical Operator/1
  Data Type Conversion/1 -> Con/1
  Compare To Constant/1 -> S-R Flip-Flop/1
  Demux/2 -> Terminator/1
  Demux/3 -> Terminator1/1
  Constant/1 -> S-R Flip-Flop/2
  S-R Flip-Flop/1 -> Terminator2/1
  S-R Flip-Flop/2 -> Logical Operator/2

== system power_aircraft_distribution/Secondary Distribution (circuit breakers)/Contactor ==
  com : Inport
  Ideal Switch : powerlib/Power Electronics/Ideal Switch  Ron=0.001  Lon=0  IC=0  Rs=1e3  Cs=inf  Measurements=off
  Ideal Switch1 : powerlib/Power Electronics/Ideal Switch  Ron=0.001  Lon=0  IC=0  Rs=1e3  Cs=inf  Measurements=off
  Ideal Switch2 : powerlib/Power Electronics/Ideal Switch  Ron=0.001  Lon=0  IC=0  Rs=1e3  Cs=inf  Measurements=off
  A : PMIOPort  Port=1  Side=Left
  a : PMIOPort  Port=2  Side=Right
  B : PMIOPort  Port=3  Side=Left
  b : PMIOPort  Port=4  Side=Right
  C : PMIOPort  Port=5  Side=Left
  c : PMIOPort  Port=6  Side=Right
  wires:
  com/1 -> Ideal Switch/1, Ideal Switch2/1, Ideal Switch1/1
  connections:
  A/RConn1 -- Ideal Switch/LConn1
  a/RConn1 -- Ideal Switch/RConn1
  B/RConn1 -- Ideal Switch1/LConn1
  b/RConn1 -- Ideal Switch1/RConn1
  C/RConn1 -- Ideal Switch2/LConn1
  c/RConn1 -- Ideal Switch2/RConn1

== system power_aircraft_distribution/Secondary Distribution (circuit breakers)/Contactor1 ==
  com : Inport
  Ideal Switch : powerlib/Power Electronics/Ideal Switch  Ron=0.001  Lon=0  IC=0  Rs=1e3  Cs=inf  Measurements=off
  Ideal Switch1 : powerlib/Power Electronics/Ideal Switch  Ron=0.001  Lon=0  IC=0  Rs=1e3  Cs=inf  Measurements=off
  Ideal Switch2 : powerlib/Power Electronics/Ideal Switch  Ron=0.001  Lon=0  IC=0  Rs=1e3  Cs=inf  Measurements=off
  A : PMIOPort  Port=1  Side=Left
  a : PMIOPort  Port=2  Side=Right
  B : PMIOPort  Port=3  Side=Left
  b : PMIOPort  Port=4  Side=Right
  C : PMIOPort  Port=5  Side=Left
  c : PMIOPort  Port=6  Side=Right
  wires:
  com/1 -> Ideal Switch1/1, Ideal Switch2/1, Ideal Switch/1
  connections:
  c/RConn1 -- Ideal Switch2/RConn1
  C/RConn1 -- Ideal Switch2/LConn1
  b/RConn1 -- Ideal Switch1/RConn1
  B/RConn1 -- Ideal Switch1/LConn1
  a/RConn1 -- Ideal Switch/RConn1
  A/RConn1 -- Ideal Switch/LConn1

== system power_aircraft_distribution/Secondary Distribution (circuit breakers)/Contactor2 ==
  com : Inport
  Ideal Switch : powerlib/Power Electronics/Ideal Switch  Ron=0.001  Lon=0  IC=0  Rs=1e3  Cs=inf  Measurements=off
  Ideal Switch1 : powerlib/Power Electronics/Ideal Switch  Ron=0.001  Lon=0  IC=0  Rs=1e3  Cs=inf  Measurements=off
  Ideal Switch2 : powerlib/Power Electronics/Ideal Switch  Ron=0.001  Lon=0  IC=0  Rs=1e3  Cs=inf  Measurements=off
  A : PMIOPort  Port=1  Side=Left
  a : PMIOPort  Port=2  Side=Right
  B : PMIOPort  Port=3  Side=Left
  b : PMIOPort  Port=4  Side=Right
  C : PMIOPort  Port=5  Side=Left
  c : PMIOPort  Port=6  Side=Right
  wires:
  com/1 -> Ideal Switch/1, Ideal Switch2/1, Ideal Switch1/1
  connections:
  A/RConn1 -- Ideal Switch/LConn1
  a/RConn1 -- Ideal Switch/RConn1
  B/RConn1 -- Ideal Switch1/LConn1
  b/RConn1 -- Ideal Switch1/RConn1
  C/RConn1 -- Ideal Switch2/LConn1
  c/RConn1 -- Ideal Switch2/RConn1

== system power_aircraft_distribution/Secondary Distribution (circuit breakers)/Contactor3 ==
  com : Inport
  Ideal Switch : powerlib/Power Electronics/Ideal Switch  Ron=0.001  Lon=0  IC=0  Rs=1e3  Cs=inf  Measurements=off
  Ideal Switch1 : powerlib/Power Electronics/Ideal Switch  Ron=0.001  Lon=0  IC=0  Rs=1e3  Cs=inf  Measurements=off
  Ideal Switch2 : powerlib/Power Electronics/Ideal Switch  Ron=0.001  Lon=0  IC=0  Rs=1e3  Cs=inf  Measurements=off
  A : PMIOPort  Port=1  Side=Left
  a : PMIOPort  Port=2  Side=Right
  B : PMIOPort  Port=3  Side=Left
  b : PMIOPort  Port=4  Side=Right
  C : PMIOPort  Port=5  Side=Left
  c : PMIOPort  Port=6  Side=Right
  wires:
  com/1 -> Ideal Switch1/1, Ideal Switch2/1, Ideal Switch/1
  connections:
  c/RConn1 -- Ideal Switch2/RConn1
  C/RConn1 -- Ideal Switch2/LConn1
  b/RConn1 -- Ideal Switch1/RConn1
  B/RConn1 -- Ideal Switch1/LConn1
  a/RConn1 -- Ideal Switch/RConn1
  A/RConn1 -- Ideal Switch/LConn1

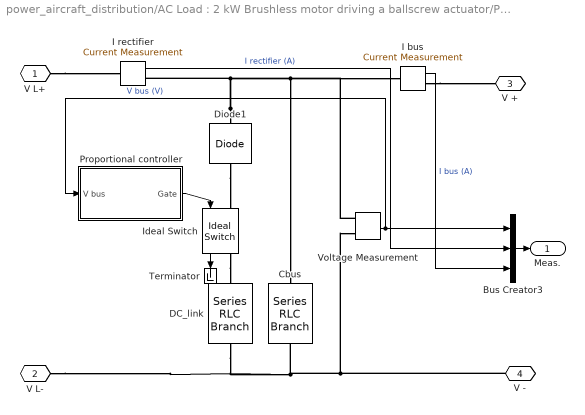
== system power_aircraft_distribution/AC Load : 2 kW Brushless motor driving a ballscrew actuator/PM Synchronous Motor Drive1/Braking chopper ==
  Bus Creator3 : BusCreator  Inputs=3
  Cbus : powerlib/Elements/Series RLC Branch  LConnTagsString=__new0  RConnTagsString=__new0  BranchType=C  Resistance=[]  Inductance=[]  SetiL0=off  InitialCurrent=0  Capacitance=cap_bus  Setx0=on  InitialVoltage=300  Measurements=None
  DC_link : powerlib/Elements/Series RLC Branch  LConnTagsString=__new0  RConnTagsString=__new0  BranchType=R  Resistance=br  Inductance=[]  SetiL0=off  InitialCurrent=0  Capacitance=[]  Setx0=off  InitialVoltage=0  Measurements=None
  Diode1 : powerlib/Power Electronics/Diode  Ron=1e-3  Lon=0  Vf=0.8  IC=0  UseSnubber=off  Rs=10e3  Cs=inf  Measurements=off
  I bus : powerlib/Measurements/Current Measurement  PhasorSimulation=off  OutputType=Complex  PSBequivalent=0
  I rectifier : powerlib/Measurements/Current Measurement  PhasorSimulation=off  OutputType=Complex  PSBequivalent=0
  Ideal Switch : powerlib/Power Electronics/Ideal Switch  Ron=1e-3  Lon=0  IC=0  Rs=10e3  Cs=inf  Measurements=on
      settings: AttributesFormatString=\n
  Proportional controller : Subsystem
  Terminator : Terminator
  Voltage Measurement : powerlib/Measurements/Voltage Measurement  Tag=PoWeRsYsTeMmEaSuReMeNt  PhasorSimulation=off  OutputType=Complex  PSBequivalent=0
  V L+ : PMIOPort  Port=1  Side=Left
  V L- : PMIOPort  Port=2  Side=Left
  V + : PMIOPort  Port=3  Side=Right
  V - : PMIOPort  Port=4  Side=Right
  Meas. : Outport
  wires:
  Ideal Switch/1 -> Terminator/1
  Voltage Measurement/1 -> Proportional controller/1(V bus), Bus Creator3/1  "V bus (V)"
  Proportional controller/1(Gate) -> Ideal Switch/1
  Bus Creator3/1 -> Meas./1
  I rectifier/1 -> Bus Creator3/2  "I rectifier (A)"
  I bus/1 -> Bus Creator3/3  "I bus (A)"
  connections:
  Ideal Switch/RConn1 -- DC_link/LConn1
  V -/RConn1 -- Voltage Measurement/LConn2 -- V L-/RConn1 -- DC_link/RConn1 -- Cbus/RConn1
  Diode1/LConn1 -- I rectifier/RConn1 -- Cbus/LConn1 -- Voltage Measurement/LConn1 -- I bus/LConn1
  Diode1/RConn1 -- Ideal Switch/LConn1
  I bus/RConn1 -- V +/RConn1
  V L+/RConn1 -- I rectifier/LConn1

== system power_aircraft_distribution/AC Load : 2 kW Brushless motor driving a ballscrew actuator/PM Synchronous Motor Drive1/Measures ==
  Current Measurement : powerlib/Measurements/Current Measurement  Tag=PoWeRsYsTeMmEaSuReMeNt  PhasorSimulation=off  OutputType=Magnitude  PSBequivalent=0
  Current Measurement1 : powerlib/Measurements/Current Measurement  Tag=PoWeRsYsTeMmEaSuReMeNt  PhasorSimulation=off  OutputType=Magnitude  PSBequivalent=0
  Current Measurement2 : powerlib/Measurements/Current Measurement  Tag=PoWeRsYsTeMmEaSuReMeNt  PhasorSimulation=off  OutputType=Magnitude  PSBequivalent=0
  Mux1 : Mux  Inputs=3
  Ta : PMIOPort  Port=1  Side=Left
  Tb : PMIOPort  Port=2  Side=Left
  Tc : PMIOPort  Port=3  Side=Left
  Mta : PMIOPort  Port=4  Side=Right
  Mtb : PMIOPort  Port=5  Side=Right
  Mtc : PMIOPort  Port=6  Side=Right
  I_abc : Outport
  wires:
  Current Measurement1/1 -> Mux1/2
  Current Measurement/1 -> Mux1/1
  Current Measurement2/1 -> Mux1/3
  Mux1/1 -> I_abc/1
  connections:
  Current Measurement1/RConn1 -- Mtb/RConn1
  Tb/RConn1 -- Current Measurement1/LConn1
  Current Measurement/RConn1 -- Mta/RConn1
  Ta/RConn1 -- Current Measurement/LConn1
  Tc/RConn1 -- Current Measurement2/LConn1
  Current Measurement2/RConn1 -- Mtc/RConn1

== system power_aircraft_distribution/AC Load : 2 kW Brushless motor driving a ballscrew actuator/PM Synchronous Motor Drive1/Braking chopper/Proportional controller ==
  V bus : Inport
  Constant : Constant  Value=chopa
  Data Type Conversion5 : DataTypeConversion  SaturateOnIntegerOverflow=on  RndMeth=Zero
  Gain : Gain  Gain=1/100  SaturateOnIntegerOverflow=on  OutDataTypeStr=Inherit: Same as input  ParamDataTypeStr=Inherit: Same as input
  Logical Operator : Logic
  Ramp_generator : Subsystem
  Relational Operator : RelationalOperator  InputSameDT=on
  Relay : Relay  OnSwitchValue=chopa  OffSwitchValue=chopd
  Sum : Sum  Inputs=|+-  SaturateOnIntegerOverflow=on  InputSameDT=on  OutDataTypeStr=Inherit: Same as first input
  Unit Delay1 : UnitDelay  SampleTime=Ts
  Gate : Outport
  wires:
  Data Type Conversion5/1 -> Logical Operator/2
  Relay/1 -> Data Type Conversion5/1
  Logical Operator/1 -> Gate/1
  Relational Operator/1 -> Logical Operator/1
  V bus/1 -> Unit Delay1/1
  Constant/1 -> Sum/2
  Gain/1 -> Relational Operator/1
  Sum/1 -> Gain/1
  Unit Delay1/1 -> Relay/1, Sum/1
  Ramp_generator/1(ramp_out) -> Relational Operator/2
